simulink model "reg_SS"  (Simulink 7.5)
settings: Solver=ode45  StartTime=0.0  StopTime=4.0  FixedStep=0.001  RelTol=1e-3
values from neighbouring files (symbols this model uses):
  c = 75    [parametri.m]
  d = 0.05    [parametri.m]
  Kda = (D2*Te^2*w02^2 - (Kw1 + Kw2)^-1*Ti*Tms*w02^2-2*zeta2*Ti*w02)/((Kw1+Kw2)^-1*Ti)    [parametri_reg.m]
  Kw1 = Tms*w02^2/w0*((2*zeta*w0*Ts+1)/(D4*D3*D2*Te*w0) - Ts*w0 - 2*zeta)    [parametri_reg.m]
  Kw2 = Ti*Tms*(1+2*zeta*w0*Ts)/(D4*D3^2*D2^3*Te^4*w0^2)-Kw1    [parametri_reg.m]
  T = pi / 10 / w0    [parametri.m]
  Tb = 1    [parametri.m]
  Tei = 2e-3    (= 0.002)    [parametri.m]
  Ti = Te - 2*zeta2/w02    [parametri_reg.m]
  Tm1 = 0.1    [parametri.m]
  Tm2 = 0.5    [parametri.m]
settings Model: Creator=Marko  LastModifiedBy=Miha
settings DebuggingCC: StrictBusMsg=Warning

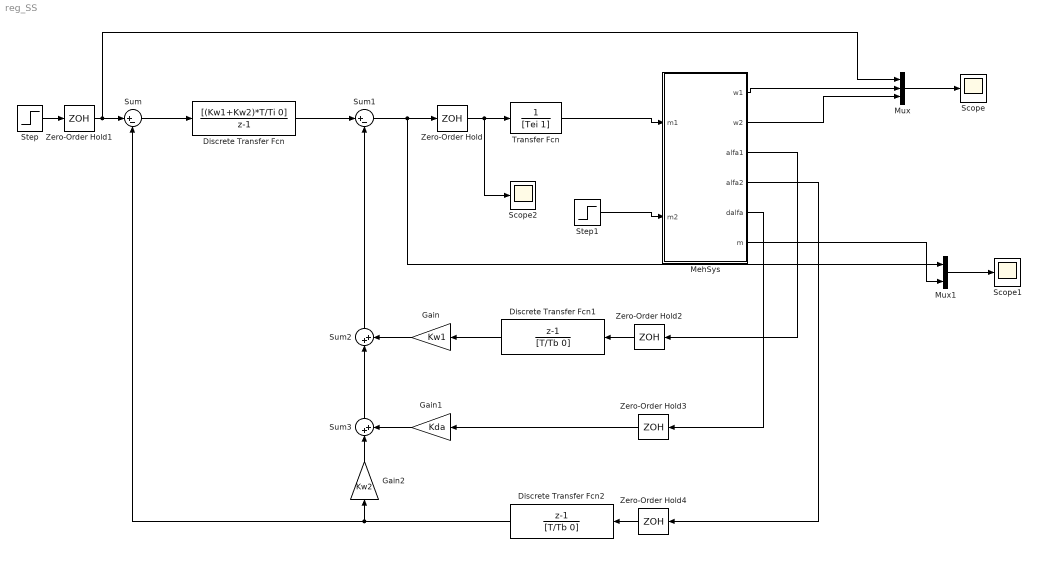
== system reg_SS ==
  Discrete Transfer Fcn : DiscreteTransferFcn  Numerator=[(Kw1+Kw2)*T/Ti 0]  Denominator=[1 -1]  SampleTime=T
  Discrete Transfer Fcn1 : DiscreteTransferFcn  Numerator=[1 -1]  Denominator=[T/Tb 0]  SampleTime=T
  Discrete Transfer Fcn2 : DiscreteTransferFcn  Numerator=[1 -1]  Denominator=[T/Tb 0]  SampleTime=T
  Gain : Gain  Gain=Kw1  ParameterDataType=fixdt(1, 16)  ParameterScaling=2^0  OutDataType=fixdt(1, 16)  OutScaling=2^0
  Gain1 : Gain  Gain=Kda  ParameterDataType=fixdt(1, 16)  ParameterScaling=2^0  OutDataType=fixdt(1, 16)  OutScaling=2^0
  Gain2 : Gain  Gain=Kw2  ParameterDataType=fixdt(1, 16)  ParameterScaling=2^0  OutDataType=fixdt(1, 16)  OutScaling=2^0
  MehSys : Subsystem
  Mux : Mux  Inputs=3
  Mux1 : Mux  Inputs=2
  Scope : Scope
      settings: SaveName=odziv_w  DataFormat=Array
  Scope1 : Scope
      settings: SaveName=odziv_m  DataFormat=Array
  Scope2 : Scope
      settings: SaveName=odziv_m1  DataFormat=Array
  Step : Step  Time=0  SampleTime=0
  Step1 : Step  Time=1.5  SampleTime=0
  Sum : Sum  Inputs=|+-  OutDataType=fixdt(1, 16)  OutScaling=2^0
  Sum1 : Sum  Inputs=|+-  OutDataType=fixdt(1, 16)  OutScaling=2^0
  Sum2 : Sum  Inputs=|++  OutDataType=fixdt(1, 16)  OutScaling=2^0
  Sum3 : Sum  Inputs=|++  OutDataType=fixdt(1, 16)  OutScaling=2^0
  Transfer Fcn : TransferFcn  Denominator=[Tei 1]
  Zero-Order Hold{,1..4} (5 alike) : ZeroOrderHold  SampleTime=T
  wires:
  MehSys/3(alfa1) -> Zero-Order Hold2/1
  MehSys/4(alfa2) -> Zero-Order Hold4/1
  Zero-Order Hold1/1 -> Sum/1, Mux/1
  Discrete Transfer Fcn/1 -> Sum1/1
  Sum1/1 -> Zero-Order Hold/1, Mux1/1
  Sum/1 -> Discrete Transfer Fcn/1
  Zero-Order Hold/1 -> Transfer Fcn/1, Scope2/1
  Transfer Fcn/1 -> MehSys/1(m1)
  Zero-Order Hold2/1 -> Discrete Transfer Fcn1/1
  Discrete Transfer Fcn1/1 -> Gain/1
  Zero-Order Hold4/1 -> Discrete Transfer Fcn2/1
  Discrete Transfer Fcn2/1 -> Sum/2, Gain2/1
  Zero-Order Hold3/1 -> Gain1/1
  Gain1/1 -> Sum3/2
  Sum3/1 -> Sum2/1
  Gain/1 -> Sum2/2
  Sum2/1 -> Sum1/2
  Step/1 -> Zero-Order Hold1/1
  Mux/1 -> Scope/1
  MehSys/5(dalfa) -> Zero-Order Hold3/1
  Step1/1 -> MehSys/2(m2)
  Gain2/1 -> Sum3/1
  MehSys/1(w1) -> Mux/2
  MehSys/2(w2) -> Mux/3
  Mux1/1 -> Scope1/1
  MehSys/6(m) -> Mux1/2

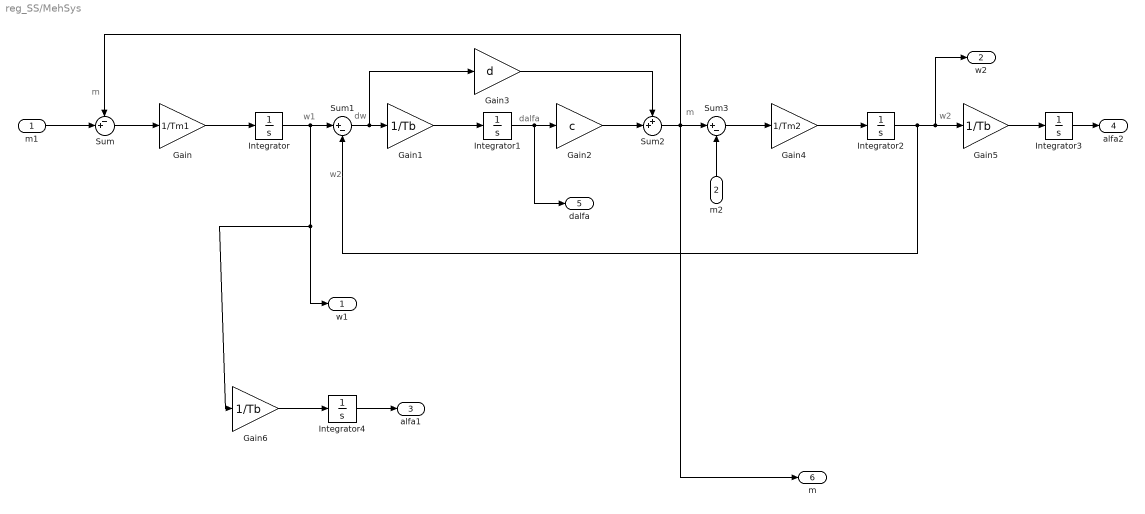
== system reg_SS/MehSys ==
  note: w2
  note: m
  note: m
  note: dalfa
  note: dw
  note: w1
  note: w2
  m1 : Inport  OutDataType=fixdt(1, 16)  OutScaling=2^0
  m2 : Inport  Port=2  OutDataType=fixdt(1, 16)  OutScaling=2^0
  Gain : Gain  Gain=1/Tm1  ParameterDataType=fixdt(1, 16)  ParameterScaling=2^0  OutDataType=fixdt(1, 16)  OutScaling=2^0
  Gain1 : Gain  Gain=1/Tb  ParameterDataType=fixdt(1, 16)  ParameterScaling=2^0  OutDataType=fixdt(1, 16)  OutScaling=2^0
  Gain2 : Gain  Gain=c  ParameterDataType=fixdt(1, 16)  ParameterScaling=2^0  OutDataType=fixdt(1, 16)  OutScaling=2^0
  Gain3 : Gain  Gain=d  ParameterDataType=fixdt(1, 16)  ParameterScaling=2^0  OutDataType=fixdt(1, 16)  OutScaling=2^0
  Gain4 : Gain  Gain=1/Tm2  ParameterDataType=fixdt(1, 16)  ParameterScaling=2^0  OutDataType=fixdt(1, 16)  OutScaling=2^0
  Gain5 : Gain  Gain=1/Tb  ParameterDataType=fixdt(1, 16)  ParameterScaling=2^0  OutDataType=fixdt(1, 16)  OutScaling=2^0
  Gain6 : Gain  Gain=1/Tb  ParameterDataType=fixdt(1, 16)  ParameterScaling=2^0  OutDataType=fixdt(1, 16)  OutScaling=2^0
  Integrator{,1..4} (5 alike) : Integrator
  Sum : Sum  Inputs=-+|  OutDataType=fixdt(1, 16)  OutScaling=2^0
  Sum1 : Sum  Inputs=|+-  OutDataType=fixdt(1, 16)  OutScaling=2^0
  Sum2 : Sum  Inputs=++|  OutDataType=fixdt(1, 16)  OutScaling=2^0
  Sum3 : Sum  Inputs=|+-  OutDataType=fixdt(1, 16)  OutScaling=2^0
  w1 : Outport  OutDataType=fixdt(1, 16)  OutScaling=2^0
  w2 : Outport  Port=2  OutDataType=fixdt(1, 16)  OutScaling=2^0
  alfa1 : Outport  Port=3  OutDataType=fixdt(1, 16)  OutScaling=2^0
  alfa2 : Outport  Port=4  OutDataType=fixdt(1, 16)  OutScaling=2^0
  dalfa : Outport  Port=5  OutDataType=fixdt(1, 16)  OutScaling=2^0
  m : Outport  Port=6  OutDataType=fixdt(1, 16)  OutScaling=2^0
  wires:
  m2/1 -> Sum3/2
  Integrator4/1 -> alfa1/1
  Gain6/1 -> Integrator4/1
  Integrator3/1 -> alfa2/1
  Gain5/1 -> Integrator3/1
  Integrator2/1 -> Sum1/2, Gain5/1, w2/1
  Gain4/1 -> Integrator2/1
  Sum3/1 -> Gain4/1
  m1/1 -> Sum/2
  Sum2/1 -> Sum3/1, Sum/1, m/1
  Gain2/1 -> Sum2/2
  Gain3/1 -> Sum2/1
  Integrator1/1 -> Gain2/1, dalfa/1
  Sum1/1 -> Gain1/1, Gain3/1
  Gain1/1 -> Integrator1/1
  Integrator/1 -> Sum1/1, w1/1, Gain6/1
  Gain/1 -> Integrator/1
  Sum/1 -> Gain/1
